simulink model "TSR_Scenario_001_cs"  (R2014b)
settings: Solver=ode5  SolverMode=SingleTasking  StartTime=0.0  StopTime=inf  FixedStep=1/100  RelTol=1e-3
PreLoadFcn:
  | mbxruntime.callbacks.PreLoadFcn(bdroot);
  | check_NUTS_defined;
  | 
  | assignin('base',['model_closed_' bdroot],false);
  | 
  | addpath('../includes_TSR/includes_TSR');
  | 
  | switch version('-release')
  | case {'2010a', '2010b', '2011a'}
  | addpath('../includes_TSR/ML2010b');
  | otherwise
  | addpath('../includes_TSR/ML2011b');
  | end
PostLoadFcn:
  | mbxruntime.callbacks.PostLoadFcn(bdroot);
InitFcn:
  | mbxruntime.callbacks.InitFcn(bdroot);
StartFcn:
  | mbxruntime.callbacks.StartFcn(bdroot);
StopFcn:
  | mbxruntime.callbacks.StopFcn(bdroot);
model workspace: external: MAT-File .\TSR_Scenario_001_cs_hws.mat (data not in the file)
undefined symbols (not defined in the file or in its folder): InitImageOutputDir, mbxruntime, OrientationPitch, OrientationRoll, PositionX, PositionY, PositionZ, tabledata, warningInitialVelocity, x0
undefined symbols (not defined in the file): SteeringColumn, SteeringWheel, TSR_Scenario_001_cs_0469e6db089af631, TSR_Scenario_001_cs_0511100212e7bc8e, TSR_Scenario_001_cs_0e7e9ae969427aac, TSR_Scenario_001_cs_1093386e49c2fe1f, TSR_Scenario_001_cs_112063adae8cf595, TSR_Scenario_001_cs_20f00d93cd5331c2, TSR_Scenario_001_cs_23e3512474fbfadc, TSR_Scenario_001_cs_366523e1554c6bf4, TSR_Scenario_001_cs_37bce4982c67337a, TSR_Scenario_001_cs_44e6164a5df50f45, TSR_Scenario_001_cs_4963ce12e7ff3247, TSR_Scenario_001_cs_4b3e01fa729ce73a, TSR_Scenario_001_cs_519c34727ce9f069, TSR_Scenario_001_cs_5b66ab60038399a1, TSR_Scenario_001_cs_5baa165dfa1afdcb, TSR_Scenario_001_cs_5f993ce39fa6372c, TSR_Scenario_001_cs_613fdf28e3ff7437, TSR_Scenario_001_cs_67b1406af835d622, TSR_Scenario_001_cs_6ad990c290286b94, TSR_Scenario_001_cs_6c412b69295984e1, TSR_Scenario_001_cs_6d4c0c06b1585ef3, TSR_Scenario_001_cs_6dd019d071bf1235, TSR_Scenario_001_cs_6e9f5883f1a78533, TSR_Scenario_001_cs_80f7223d9ac35404, TSR_Scenario_001_cs_8562b82d3c89ae57, TSR_Scenario_001_cs_8a3a0181ab0babfe, TSR_Scenario_001_cs_8c997348ce80deaf, TSR_Scenario_001_cs_925bd6a073d9fe25, TSR_Scenario_001_cs_961436216add6114, TSR_Scenario_001_cs_991a7959256b2c84, TSR_Scenario_001_cs_9a95ce2c2e753616, TSR_Scenario_001_cs_a98aa9562e8552a9, TSR_Scenario_001_cs_ab44ae81dbfb58cd, TSR_Scenario_001_cs_Actros_2541_2_Path_pathUniqueID, TSR_Scenario_001_cs_ae74836ade6bff5a, TSR_Scenario_001_cs_Audi_A8_1_Dynamics_Simple_initialPitch, TSR_Scenario_001_cs_Audi_A8_1_Dynamics_Simple_initialRoll, TSR_Scenario_001_cs_Audi_A8_1_Dynamics_Simple_initialX, TSR_Scenario_001_cs_Audi_A8_1_Dynamics_Simple_initialY, TSR_Scenario_001_cs_Audi_A8_1_Dynamics_Simple_initialYaw, TSR_Scenario_001_cs_Audi_A8_1_Dynamics_Simple_initialZ, TSR_Scenario_001_cs_Audi_A8_2_Path_pathUniqueID, TSR_Scenario_001_cs_Audi_A8_2_SpeedProfile_speedProfileUniqueID, TSR_Scenario_001_cs_b2eca4eb2fce349a, TSR_Scenario_001_cs_b7bac209c1f2549f, TSR_Scenario_001_cs_bf3dccb66d3255a4, TSR_Scenario_001_cs_bf4c1a5315e3f716, TSR_Scenario_001_cs_BMW_Z3_1_Path_pathUniqueID, TSR_Scenario_001_cs_BMW_Z3_1_SpeedProfile_speedProfileUniqueID, TSR_Scenario_001_cs_BMW_Z3_2_Path_pathUniqueID, TSR_Scenario_001_cs_BMW_Z3_2_SpeedProfile_speedProfileUniqueID, TSR_Scenario_001_cs_c4c8fc4bdece03a9, TSR_Scenario_001_cs_c964c86aa54ad92e, TSR_Scenario_001_cs_cb64d1ef85329755, TSR_Scenario_001_cs_Citroen_C3_1_Path_pathUniqueID, TSR_Scenario_001_cs_Citroen_C3_2_Path_pathUniqueID, TSR_Scenario_001_cs_Citroen_C3_3_Path_pathUniqueID, TSR_Scenario_001_cs_Citroen_C3_4_Path_pathUniqueID ... (+25)
libraries: simulink x21, PreScanSimulinkLibrary x17, simulink_extras x13
(part 16 of 30)

== system TSR_Scenario_001_cs/VISUMatrixSignLights_HighwayOverhang_6/Actuator ==
  VISUMatrixSignLights_HighwayOverhang_6 : Inport  Tag=inport/VisuMatrixSignLights  SampleTime=1/100  BusOutputAsStruct=on
  DemuxVisuLights : Demux  Outputs=16
  LimiterVisuLights : Saturate  UpperLimit=1  LowerLimit=0
  visu_MatrixSign_21_Light_1 : S-Function  FunctionName=sfun_MaterialColorSelector  Parameters=mbxruntime.parameters.convert(UniqueID), mbxruntime.parameters.convert(ColorsObjectQuery), mbxruntime.parameters.convert(Colors),tabledata, TimeStep  EnableBusSupport=off  mask(PreScan Sink Block: VisuMatrixSignLights){UniqueID=1914, ColorsObjectQuery=child:name=MatrixSign_21/child:name=HighwayOverhang_6.MatrixSign_21.OrangeLightUpperLeft, Colors=[32   25    5  255   64   48    5  255   64   54    5  255    0    0    0  255; 45   34    0  255   45   34    0  255   45   34    0  255  306  229    5  255], TimeStep=1/100}
      mask prompts: UniqueID "Parent Unique Identifier"; ColorsObjectQuery "Query for Color Object"; Colors "Matrix of colors"; TimeStep "Simulink time step"
      mask help:
      | The VisuMatrixSignLights block provides a way to switch the lights on the matrix sign board on or off
      |
      | For more information, please click Help.
      mask init:
      | [tabledata] = mbxruntime.parameters.table(UniqueID,ColorsObjectQuery,Colors);
      mask Help: eval('openHelp(732)')
      mask Display: image(imread('RearLight.png'))
  visu_MatrixSign_21_Light_2 : S-Function  FunctionName=sfun_MaterialColorSelector  Parameters=mbxruntime.parameters.convert(UniqueID), mbxruntime.parameters.convert(ColorsObjectQuery), mbxruntime.parameters.convert(Colors),tabledata, TimeStep  EnableBusSupport=off  mask(PreScan Sink Block: VisuMatrixSignLights){UniqueID=1914, ColorsObjectQuery=child:name=MatrixSign_21/child:name=HighwayOverhang_6.MatrixSign_21.OrangeLightUpperRight, Colors=[32   25    5  255   64   48    5  255   64   54    5  255    0    0    0  255; 45   34    0  255   45   34    0  255   45   34    0  255  306  229    5  255], TimeStep=1/100}
      mask prompts: UniqueID "Parent Unique Identifier"; ColorsObjectQuery "Query for Color Object"; Colors "Matrix of colors"; TimeStep "Simulink time step"
      mask help:
      | The VisuMatrixSignLights block provides a way to switch the lights on the matrix sign board on or off
      |
      | For more information, please click Help.
      mask init:
      | [tabledata] = mbxruntime.parameters.table(UniqueID,ColorsObjectQuery,Colors);
      mask Help: eval('openHelp(732)')
      mask Display: image(imread('RearLight.png'))
  visu_MatrixSign_21_Light_3 : S-Function  FunctionName=sfun_MaterialColorSelector  Parameters=mbxruntime.parameters.convert(UniqueID), mbxruntime.parameters.convert(ColorsObjectQuery), mbxruntime.parameters.convert(Colors),tabledata, TimeStep  EnableBusSupport=off  mask(PreScan Sink Block: VisuMatrixSignLights){UniqueID=1914, ColorsObjectQuery=child:name=MatrixSign_21/child:name=HighwayOverhang_6.MatrixSign_21.OrangeLightLowerLeft, Colors=[32   25    5  255   64   48    5  255   64   54    5  255    0    0    0  255; 45   34    0  255   45   34    0  255   45   34    0  255  306  229    5  255], TimeStep=1/100}
      mask prompts: UniqueID "Parent Unique Identifier"; ColorsObjectQuery "Query for Color Object"; Colors "Matrix of colors"; TimeStep "Simulink time step"
      mask help:
      | The VisuMatrixSignLights block provides a way to switch the lights on the matrix sign board on or off
      |
      | For more information, please click Help.
      mask init:
      | [tabledata] = mbxruntime.parameters.table(UniqueID,ColorsObjectQuery,Colors);
      mask Help: eval('openHelp(732)')
      mask Display: image(imread('RearLight.png'))
  visu_MatrixSign_21_Light_4 : S-Function  FunctionName=sfun_MaterialColorSelector  Parameters=mbxruntime.parameters.convert(UniqueID), mbxruntime.parameters.convert(ColorsObjectQuery), mbxruntime.parameters.convert(Colors),tabledata, TimeStep  EnableBusSupport=off  mask(PreScan Sink Block: VisuMatrixSignLights){UniqueID=1914, ColorsObjectQuery=child:name=MatrixSign_21/child:name=HighwayOverhang_6.MatrixSign_21.OrangeLightLowerRight, Colors=[32   25    5  255   64   48    5  255   64   54    5  255    0    0    0  255; 45   34    0  255   45   34    0  255   45   34    0  255  306  229    5  255], TimeStep=1/100}
      mask prompts: UniqueID "Parent Unique Identifier"; ColorsObjectQuery "Query for Color Object"; Colors "Matrix of colors"; TimeStep "Simulink time step"
      mask help:
      | The VisuMatrixSignLights block provides a way to switch the lights on the matrix sign board on or off
      |
      | For more information, please click Help.
      mask init:
      | [tabledata] = mbxruntime.parameters.table(UniqueID,ColorsObjectQuery,Colors);
      mask Help: eval('openHelp(732)')
      mask Display: image(imread('RearLight.png'))
  visu_MatrixSign_22_Light_1 : S-Function  FunctionName=sfun_MaterialColorSelector  Parameters=mbxruntime.parameters.convert(UniqueID), mbxruntime.parameters.convert(ColorsObjectQuery), mbxruntime.parameters.convert(Colors),tabledata, TimeStep  EnableBusSupport=off  mask(PreScan Sink Block: VisuMatrixSignLights){UniqueID=1914, ColorsObjectQuery=child:name=MatrixSign_22/child:name=HighwayOverhang_6.MatrixSign_22.OrangeLightUpperLeft, Colors=[32   25    5  255   64   48    5  255   64   54    5  255    0    0    0  255; 45   34    0  255   45   34    0  255   45   34    0  255  306  229    5  255], TimeStep=1/100}
      mask prompts: UniqueID "Parent Unique Identifier"; ColorsObjectQuery "Query for Color Object"; Colors "Matrix of colors"; TimeStep "Simulink time step"
      mask help:
      | The VisuMatrixSignLights block provides a way to switch the lights on the matrix sign board on or off
      |
      | For more information, please click Help.
      mask init:
      | [tabledata] = mbxruntime.parameters.table(UniqueID,ColorsObjectQuery,Colors);
      mask Help: eval('openHelp(732)')
      mask Display: image(imread('RearLight.png'))
  visu_MatrixSign_22_Light_2 : S-Function  FunctionName=sfun_MaterialColorSelector  Parameters=mbxruntime.parameters.convert(UniqueID), mbxruntime.parameters.convert(ColorsObjectQuery), mbxruntime.parameters.convert(Colors),tabledata, TimeStep  EnableBusSupport=off  mask(PreScan Sink Block: VisuMatrixSignLights){UniqueID=1914, ColorsObjectQuery=child:name=MatrixSign_22/child:name=HighwayOverhang_6.MatrixSign_22.OrangeLightUpperRight, Colors=[32   25    5  255   64   48    5  255   64   54    5  255    0    0    0  255; 45   34    0  255   45   34    0  255   45   34    0  255  306  229    5  255], TimeStep=1/100}
      mask prompts: UniqueID "Parent Unique Identifier"; ColorsObjectQuery "Query for Color Object"; Colors "Matrix of colors"; TimeStep "Simulink time step"
      mask help:
      | The VisuMatrixSignLights block provides a way to switch the lights on the matrix sign board on or off
      |
      | For more information, please click Help.
      mask init:
      | [tabledata] = mbxruntime.parameters.table(UniqueID,ColorsObjectQuery,Colors);
      mask Help: eval('openHelp(732)')
      mask Display: image(imread('RearLight.png'))
  visu_MatrixSign_22_Light_3 : S-Function  FunctionName=sfun_MaterialColorSelector  Parameters=mbxruntime.parameters.convert(UniqueID), mbxruntime.parameters.convert(ColorsObjectQuery), mbxruntime.parameters.convert(Colors),tabledata, TimeStep  EnableBusSupport=off  mask(PreScan Sink Block: VisuMatrixSignLights){UniqueID=1914, ColorsObjectQuery=child:name=MatrixSign_22/child:name=HighwayOverhang_6.MatrixSign_22.OrangeLightLowerLeft, Colors=[32   25    5  255   64   48    5  255   64   54    5  255    0    0    0  255; 45   34    0  255   45   34    0  255   45   34    0  255  306  229    5  255], TimeStep=1/100}
      mask prompts: UniqueID "Parent Unique Identifier"; ColorsObjectQuery "Query for Color Object"; Colors "Matrix of colors"; TimeStep "Simulink time step"
      mask help:
      | The VisuMatrixSignLights block provides a way to switch the lights on the matrix sign board on or off
      |
      | For more information, please click Help.
      mask init:
      | [tabledata] = mbxruntime.parameters.table(UniqueID,ColorsObjectQuery,Colors);
      mask Help: eval('openHelp(732)')
      mask Display: image(imread('RearLight.png'))
  visu_MatrixSign_22_Light_4 : S-Function  FunctionName=sfun_MaterialColorSelector  Parameters=mbxruntime.parameters.convert(UniqueID), mbxruntime.parameters.convert(ColorsObjectQuery), mbxruntime.parameters.convert(Colors),tabledata, TimeStep  EnableBusSupport=off  mask(PreScan Sink Block: VisuMatrixSignLights){UniqueID=1914, ColorsObjectQuery=child:name=MatrixSign_22/child:name=HighwayOverhang_6.MatrixSign_22.OrangeLightLowerRight, Colors=[32   25    5  255   64   48    5  255   64   54    5  255    0    0    0  255; 45   34    0  255   45   34    0  255   45   34    0  255  306  229    5  255], TimeStep=1/100}
      mask prompts: UniqueID "Parent Unique Identifier"; ColorsObjectQuery "Query for Color Object"; Colors "Matrix of colors"; TimeStep "Simulink time step"
      mask help:
      | The VisuMatrixSignLights block provides a way to switch the lights on the matrix sign board on or off
      |
      | For more information, please click Help.
      mask init:
      | [tabledata] = mbxruntime.parameters.table(UniqueID,ColorsObjectQuery,Colors);
      mask Help: eval('openHelp(732)')
      mask Display: image(imread('RearLight.png'))
  visu_MatrixSign_23_Light_1 : S-Function  FunctionName=sfun_MaterialColorSelector  Parameters=mbxruntime.parameters.convert(UniqueID), mbxruntime.parameters.convert(ColorsObjectQuery), mbxruntime.parameters.convert(Colors),tabledata, TimeStep  EnableBusSupport=off  mask(PreScan Sink Block: VisuMatrixSignLights){UniqueID=1914, ColorsObjectQuery=child:name=MatrixSign_23/child:name=HighwayOverhang_6.MatrixSign_23.OrangeLightUpperLeft, Colors=[32   25    5  255   64   48    5  255   64   54    5  255    0    0    0  255; 45   34    0  255   45   34    0  255   45   34    0  255  306  229    5  255], TimeStep=1/100}
      mask prompts: UniqueID "Parent Unique Identifier"; ColorsObjectQuery "Query for Color Object"; Colors "Matrix of colors"; TimeStep "Simulink time step"
      mask help:
      | The VisuMatrixSignLights block provides a way to switch the lights on the matrix sign board on or off
      |
      | For more information, please click Help.
      mask init:
      | [tabledata] = mbxruntime.parameters.table(UniqueID,ColorsObjectQuery,Colors);
      mask Help: eval('openHelp(732)')
      mask Display: image(imread('RearLight.png'))
  visu_MatrixSign_23_Light_2 : S-Function  FunctionName=sfun_MaterialColorSelector  Parameters=mbxruntime.parameters.convert(UniqueID), mbxruntime.parameters.convert(ColorsObjectQuery), mbxruntime.parameters.convert(Colors),tabledata, TimeStep  EnableBusSupport=off  mask(PreScan Sink Block: VisuMatrixSignLights){UniqueID=1914, ColorsObjectQuery=child:name=MatrixSign_23/child:name=HighwayOverhang_6.MatrixSign_23.OrangeLightUpperRight, Colors=[32   25    5  255   64   48    5  255   64   54    5  255    0    0    0  255; 45   34    0  255   45   34    0  255   45   34    0  255  306  229    5  255], TimeStep=1/100}
      mask prompts: UniqueID "Parent Unique Identifier"; ColorsObjectQuery "Query for Color Object"; Colors "Matrix of colors"; TimeStep "Simulink time step"
      mask help:
      | The VisuMatrixSignLights block provides a way to switch the lights on the matrix sign board on or off
      |
      | For more information, please click Help.
      mask init:
      | [tabledata] = mbxruntime.parameters.table(UniqueID,ColorsObjectQuery,Colors);
      mask Help: eval('openHelp(732)')
      mask Display: image(imread('RearLight.png'))
  visu_MatrixSign_23_Light_3 : S-Function  FunctionName=sfun_MaterialColorSelector  Parameters=mbxruntime.parameters.convert(UniqueID), mbxruntime.parameters.convert(ColorsObjectQuery), mbxruntime.parameters.convert(Colors),tabledata, TimeStep  EnableBusSupport=off  mask(PreScan Sink Block: VisuMatrixSignLights){UniqueID=1914, ColorsObjectQuery=child:name=MatrixSign_23/child:name=HighwayOverhang_6.MatrixSign_23.OrangeLightLowerLeft, Colors=[32   25    5  255   64   48    5  255   64   54    5  255    0    0    0  255; 45   34    0  255   45   34    0  255   45   34    0  255  306  229    5  255], TimeStep=1/100}
      mask prompts: UniqueID "Parent Unique Identifier"; ColorsObjectQuery "Query for Color Object"; Colors "Matrix of colors"; TimeStep "Simulink time step"
      mask help:
      | The VisuMatrixSignLights block provides a way to switch the lights on the matrix sign board on or off
      |
      | For more information, please click Help.
      mask init:
      | [tabledata] = mbxruntime.parameters.table(UniqueID,ColorsObjectQuery,Colors);
      mask Help: eval('openHelp(732)')
      mask Display: image(imread('RearLight.png'))
  visu_MatrixSign_23_Light_4 : S-Function  FunctionName=sfun_MaterialColorSelector  Parameters=mbxruntime.parameters.convert(UniqueID), mbxruntime.parameters.convert(ColorsObjectQuery), mbxruntime.parameters.convert(Colors),tabledata, TimeStep  EnableBusSupport=off  mask(PreScan Sink Block: VisuMatrixSignLights){UniqueID=1914, ColorsObjectQuery=child:name=MatrixSign_23/child:name=HighwayOverhang_6.MatrixSign_23.OrangeLightLowerRight, Colors=[32   25    5  255   64   48    5  255   64   54    5  255    0    0    0  255; 45   34    0  255   45   34    0  255   45   34    0  255  306  229    5  255], TimeStep=1/100}
      mask prompts: UniqueID "Parent Unique Identifier"; ColorsObjectQuery "Query for Color Object"; Colors "Matrix of colors"; TimeStep "Simulink time step"
      mask help:
      | The VisuMatrixSignLights block provides a way to switch the lights on the matrix sign board on or off
      |
      | For more information, please click Help.
      mask init:
      | [tabledata] = mbxruntime.parameters.table(UniqueID,ColorsObjectQuery,Colors);
      mask Help: eval('openHelp(732)')
      mask Display: image(imread('RearLight.png'))
  visu_MatrixSign_24_Light_1 : S-Function  FunctionName=sfun_MaterialColorSelector  Parameters=mbxruntime.parameters.convert(UniqueID), mbxruntime.parameters.convert(ColorsObjectQuery), mbxruntime.parameters.convert(Colors),tabledata, TimeStep  EnableBusSupport=off  mask(PreScan Sink Block: VisuMatrixSignLights){UniqueID=1914, ColorsObjectQuery=child:name=MatrixSign_24/child:name=HighwayOverhang_6.MatrixSign_24.OrangeLightUpperLeft, Colors=[32   25    5  255   64   48    5  255   64   54    5  255    0    0    0  255; 45   34    0  255   45   34    0  255   45   34    0  255  306  229    5  255], TimeStep=1/100}
      mask prompts: UniqueID "Parent Unique Identifier"; ColorsObjectQuery "Query for Color Object"; Colors "Matrix of colors"; TimeStep "Simulink time step"
      mask help:
      | The VisuMatrixSignLights block provides a way to switch the lights on the matrix sign board on or off
      |
      | For more information, please click Help.
      mask init:
      | [tabledata] = mbxruntime.parameters.table(UniqueID,ColorsObjectQuery,Colors);
      mask Help: eval('openHelp(732)')
      mask Display: image(imread('RearLight.png'))
  visu_MatrixSign_24_Light_2 : S-Function  FunctionName=sfun_MaterialColorSelector  Parameters=mbxruntime.parameters.convert(UniqueID), mbxruntime.parameters.convert(ColorsObjectQuery), mbxruntime.parameters.convert(Colors),tabledata, TimeStep  EnableBusSupport=off  mask(PreScan Sink Block: VisuMatrixSignLights){UniqueID=1914, ColorsObjectQuery=child:name=MatrixSign_24/child:name=HighwayOverhang_6.MatrixSign_24.OrangeLightUpperRight, Colors=[32   25    5  255   64   48    5  255   64   54    5  255    0    0    0  255; 45   34    0  255   45   34    0  255   45   34    0  255  306  229    5  255], TimeStep=1/100}
      mask prompts: UniqueID "Parent Unique Identifier"; ColorsObjectQuery "Query for Color Object"; Colors "Matrix of colors"; TimeStep "Simulink time step"
      mask help:
      | The VisuMatrixSignLights block provides a way to switch the lights on the matrix sign board on or off
      |
      | For more information, please click Help.
      mask init:
      | [tabledata] = mbxruntime.parameters.table(UniqueID,ColorsObjectQuery,Colors);
      mask Help: eval('openHelp(732)')
      mask Display: image(imread('RearLight.png'))
  visu_MatrixSign_24_Light_3 : S-Function  FunctionName=sfun_MaterialColorSelector  Parameters=mbxruntime.parameters.convert(UniqueID), mbxruntime.parameters.convert(ColorsObjectQuery), mbxruntime.parameters.convert(Colors),tabledata, TimeStep  EnableBusSupport=off  mask(PreScan Sink Block: VisuMatrixSignLights){UniqueID=1914, ColorsObjectQuery=child:name=MatrixSign_24/child:name=HighwayOverhang_6.MatrixSign_24.OrangeLightLowerLeft, Colors=[32   25    5  255   64   48    5  255   64   54    5  255    0    0    0  255; 45   34    0  255   45   34    0  255   45   34    0  255  306  229    5  255], TimeStep=1/100}
      mask prompts: UniqueID "Parent Unique Identifier"; ColorsObjectQuery "Query for Color Object"; Colors "Matrix of colors"; TimeStep "Simulink time step"
      mask help:
      | The VisuMatrixSignLights block provides a way to switch the lights on the matrix sign board on or off
      |
      | For more information, please click Help.
      mask init:
      | [tabledata] = mbxruntime.parameters.table(UniqueID,ColorsObjectQuery,Colors);
      mask Help: eval('openHelp(732)')
      mask Display: image(imread('RearLight.png'))
  visu_MatrixSign_24_Light_4 : S-Function  FunctionName=sfun_MaterialColorSelector  Parameters=mbxruntime.parameters.convert(UniqueID), mbxruntime.parameters.convert(ColorsObjectQuery), mbxruntime.parameters.convert(Colors),tabledata, TimeStep  EnableBusSupport=off  mask(PreScan Sink Block: VisuMatrixSignLights){UniqueID=1914, ColorsObjectQuery=child:name=MatrixSign_24/child:name=HighwayOverhang_6.MatrixSign_24.OrangeLightLowerRight, Colors=[32   25    5  255   64   48    5  255   64   54    5  255    0    0    0  255; 45   34    0  255   45   34    0  255   45   34    0  255  306  229    5  255], TimeStep=1/100}
      mask prompts: UniqueID "Parent Unique Identifier"; ColorsObjectQuery "Query for Color Object"; Colors "Matrix of colors"; TimeStep "Simulink time step"
      mask help:
      | The VisuMatrixSignLights block provides a way to switch the lights on the matrix sign board on or off
      |
      | For more information, please click Help.
      mask init:
      | [tabledata] = mbxruntime.parameters.table(UniqueID,ColorsObjectQuery,Colors);
      mask Help: eval('openHelp(732)')
      mask Display: image(imread('RearLight.png'))
  wires:
  VISUMatrixSignLights_HighwayOverhang_6/1 -> LimiterVisuLights/1
  LimiterVisuLights/1 -> DemuxVisuLights/1
  DemuxVisuLights/1 -> visu_MatrixSign_21_Light_1/1
  DemuxVisuLights/2 -> visu_MatrixSign_21_Light_2/1
  DemuxVisuLights/3 -> visu_MatrixSign_21_Light_3/1
  DemuxVisuLights/4 -> visu_MatrixSign_21_Light_4/1
  DemuxVisuLights/5 -> visu_MatrixSign_22_Light_1/1
  DemuxVisuLights/6 -> visu_MatrixSign_22_Light_2/1
  DemuxVisuLights/7 -> visu_MatrixSign_22_Light_3/1
  DemuxVisuLights/8 -> visu_MatrixSign_22_Light_4/1
  DemuxVisuLights/9 -> visu_MatrixSign_23_Light_1/1
  DemuxVisuLights/10 -> visu_MatrixSign_23_Light_2/1
  DemuxVisuLights/11 -> visu_MatrixSign_23_Light_3/1
  DemuxVisuLights/12 -> visu_MatrixSign_23_Light_4/1
  DemuxVisuLights/13 -> visu_MatrixSign_24_Light_1/1
  DemuxVisuLights/14 -> visu_MatrixSign_24_Light_2/1
  DemuxVisuLights/15 -> visu_MatrixSign_24_Light_3/1
  DemuxVisuLights/16 -> visu_MatrixSign_24_Light_4/1

== system TSR_Scenario_001_cs/VISUMatrixSign_HighwayOverhang_1/Actuator ==
  VISUMatrixSign_HighwayOverhang_1 : Inport  Tag=inport/VisuMatrixSign  SampleTime=1/100  BusOutputAsStruct=on
  DemuxVisuMatrixSign : Demux
  visu_MatrixSign_1 : S-Function  FunctionName=sfun_ResourceNameSelector  Parameters=mbxruntime.parameters.convert(UniqueID), mbxruntime.parameters.convert(ResourceList), mbxruntime.parameters.convert(PivotName),tabledata, TimeStep  EnableBusSupport=off  mask(PreScan Sink Block: VisuMatrixSign){UniqueID=1876, ResourceList={'3' 'InformationSign\MatrixSign_Empty.png' '4' 'InformationSign\MatrixSign_End.png' '5' 'InformationSign\MatrixSign_GreenArrow.png' '6' 'InformationSign\MatrixSign_RedCross.png' '7' 'InformationSign\MatrixSign_Speed_50.png' '8' 'InformationSign\MatrixSign_Speed_70.png' '9' 'InformationSign\MatrixSign_Speed_90.png' '10' 'InformationSign\MatrixSign_Speed_120.png' '11' 'InformationSign\MatrixSign_Speed_130.png' '12' 'InformationSign\information.png' '13' 'InformationSign\Empty.jpg' }, PivotName=/child:name=MatrixSign_1/trafficSignElement, TimeStep=1/100}
      mask prompts: UniqueID "Parent Unique Identifier (auto-generated)"; ResourceList "Resource List (auto-generated)"; PivotName "Name of pivot (auto-generated)"; TimeStep "Simulink time step"
      mask help:
      | The VisuMatrixSign block provides a way to adapt the texture of the plates connected to an overhang, based on Resource IDs of the texture files.
      |
      | For more information, please click Help.
      mask init:
      | [tabledata] = mbxruntime.parameters.table(UniqueID,ResourceList,PivotName);
      mask Help: eval('openHelp(733)')
      mask Display: image(imread('HighwaySpeedMatrix.png'))
  visu_MatrixSign_2 : S-Function  FunctionName=sfun_ResourceNameSelector  Parameters=mbxruntime.parameters.convert(UniqueID), mbxruntime.parameters.convert(ResourceList), mbxruntime.parameters.convert(PivotName),tabledata, TimeStep  EnableBusSupport=off  mask(PreScan Sink Block: VisuMatrixSign){UniqueID=1876, ResourceList={'3' 'InformationSign\MatrixSign_Empty.png' '4' 'InformationSign\MatrixSign_End.png' '5' 'InformationSign\MatrixSign_GreenArrow.png' '6' 'InformationSign\MatrixSign_RedCross.png' '7' 'InformationSign\MatrixSign_Speed_50.png' '8' 'InformationSign\MatrixSign_Speed_70.png' '9' 'InformationSign\MatrixSign_Speed_90.png' '10' 'InformationSign\MatrixSign_Speed_120.png' '11' 'InformationSign\MatrixSign_Speed_130.png' '12' 'InformationSign\information.png' '13' 'InformationSign\Empty.jpg' }, PivotName=/child:name=MatrixSign_2/trafficSignElement, TimeStep=1/100}
      mask prompts: UniqueID "Parent Unique Identifier (auto-generated)"; ResourceList "Resource List (auto-generated)"; PivotName "Name of pivot (auto-generated)"; TimeStep "Simulink time step"
      mask help:
      | The VisuMatrixSign block provides a way to adapt the texture of the plates connected to an overhang, based on Resource IDs of the texture files.
      |
      | For more information, please click Help.
      mask init:
      | [tabledata] = mbxruntime.parameters.table(UniqueID,ResourceList,PivotName);
      mask Help: eval('openHelp(733)')
      mask Display: image(imread('HighwaySpeedMatrix.png'))
  visu_MatrixSign_3 : S-Function  FunctionName=sfun_ResourceNameSelector  Parameters=mbxruntime.parameters.convert(UniqueID), mbxruntime.parameters.convert(ResourceList), mbxruntime.parameters.convert(PivotName),tabledata, TimeStep  EnableBusSupport=off  mask(PreScan Sink Block: VisuMatrixSign){UniqueID=1876, ResourceList={'3' 'InformationSign\MatrixSign_Empty.png' '4' 'InformationSign\MatrixSign_End.png' '5' 'InformationSign\MatrixSign_GreenArrow.png' '6' 'InformationSign\MatrixSign_RedCross.png' '7' 'InformationSign\MatrixSign_Speed_50.png' '8' 'InformationSign\MatrixSign_Speed_70.png' '9' 'InformationSign\MatrixSign_Speed_90.png' '10' 'InformationSign\MatrixSign_Speed_120.png' '11' 'InformationSign\MatrixSign_Speed_130.png' '12' 'InformationSign\information.png' '13' 'InformationSign\Empty.jpg' }, PivotName=/child:name=MatrixSign_3/trafficSignElement, TimeStep=1/100}
      mask prompts: UniqueID "Parent Unique Identifier (auto-generated)"; ResourceList "Resource List (auto-generated)"; PivotName "Name of pivot (auto-generated)"; TimeStep "Simulink time step"
      mask help:
      | The VisuMatrixSign block provides a way to adapt the texture of the plates connected to an overhang, based on Resource IDs of the texture files.
      |
      | For more information, please click Help.
      mask init:
      | [tabledata] = mbxruntime.parameters.table(UniqueID,ResourceList,PivotName);
      mask Help: eval('openHelp(733)')
      mask Display: image(imread('HighwaySpeedMatrix.png'))
  visu_MatrixSign_4 : S-Function  FunctionName=sfun_ResourceNameSelector  Parameters=mbxruntime.parameters.convert(UniqueID), mbxruntime.parameters.convert(ResourceList), mbxruntime.parameters.convert(PivotName),tabledata, TimeStep  EnableBusSupport=off  mask(PreScan Sink Block: VisuMatrixSign){UniqueID=1876, ResourceList={'3' 'InformationSign\MatrixSign_Empty.png' '4' 'InformationSign\MatrixSign_End.png' '5' 'InformationSign\MatrixSign_GreenArrow.png' '6' 'InformationSign\MatrixSign_RedCross.png' '7' 'InformationSign\MatrixSign_Speed_50.png' '8' 'InformationSign\MatrixSign_Speed_70.png' '9' 'InformationSign\MatrixSign_Speed_90.png' '10' 'InformationSign\MatrixSign_Speed_120.png' '11' 'InformationSign\MatrixSign_Speed_130.png' '12' 'InformationSign\information.png' '13' 'InformationSign\Empty.jpg' }, PivotName=/child:name=MatrixSign_4/trafficSignElement, TimeStep=1/100}
      mask prompts: UniqueID "Parent Unique Identifier (auto-generated)"; ResourceList "Resource List (auto-generated)"; PivotName "Name of pivot (auto-generated)"; TimeStep "Simulink time step"
      mask help:
      | The VisuMatrixSign block provides a way to adapt the texture of the plates connected to an overhang, based on Resource IDs of the texture files.
      |
      | For more information, please click Help.
      mask init:
      | [tabledata] = mbxruntime.parameters.table(UniqueID,ResourceList,PivotName);
      mask Help: eval('openHelp(733)')
      mask Display: image(imread('HighwaySpeedMatrix.png'))
  wires:
  VISUMatrixSign_HighwayOverhang_1/1 -> DemuxVisuMatrixSign/1
  DemuxVisuMatrixSign/1 -> visu_MatrixSign_1/1
  DemuxVisuMatrixSign/2 -> visu_MatrixSign_2/1
  DemuxVisuMatrixSign/3 -> visu_MatrixSign_3/1
  DemuxVisuMatrixSign/4 -> visu_MatrixSign_4/1

== system TSR_Scenario_001_cs/VISUMatrixSign_HighwayOverhang_2/Actuator ==
  VISUMatrixSign_HighwayOverhang_2 : Inport  Tag=inport/VisuMatrixSign  SampleTime=1/100  BusOutputAsStruct=on
  DemuxVisuMatrixSign : Demux
  visu_MatrixSign_5 : S-Function  FunctionName=sfun_ResourceNameSelector  Parameters=mbxruntime.parameters.convert(UniqueID), mbxruntime.parameters.convert(ResourceList), mbxruntime.parameters.convert(PivotName),tabledata, TimeStep  EnableBusSupport=off  mask(PreScan Sink Block: VisuMatrixSign){UniqueID=1877, ResourceList={'3' 'InformationSign\MatrixSign_Empty.png' '4' 'InformationSign\MatrixSign_End.png' '5' 'InformationSign\MatrixSign_GreenArrow.png' '6' 'InformationSign\MatrixSign_RedCross.png' '7' 'InformationSign\MatrixSign_Speed_50.png' '8' 'InformationSign\MatrixSign_Speed_70.png' '9' 'InformationSign\MatrixSign_Speed_90.png' '10' 'InformationSign\MatrixSign_Speed_120.png' '11' 'InformationSign\MatrixSign_Speed_130.png' '12' 'InformationSign\information.png' '13' 'InformationSign\Empty.jpg' }, PivotName=/child:name=MatrixSign_5/trafficSignElement, TimeStep=1/100}
      mask prompts: UniqueID "Parent Unique Identifier (auto-generated)"; ResourceList "Resource List (auto-generated)"; PivotName "Name of pivot (auto-generated)"; TimeStep "Simulink time step"
      mask help:
      | The VisuMatrixSign block provides a way to adapt the texture of the plates connected to an overhang, based on Resource IDs of the texture files.
      |
      | For more information, please click Help.
      mask init:
      | [tabledata] = mbxruntime.parameters.table(UniqueID,ResourceList,PivotName);
      mask Help: eval('openHelp(733)')
      mask Display: image(imread('HighwaySpeedMatrix.png'))
  visu_MatrixSign_6 : S-Function  FunctionName=sfun_ResourceNameSelector  Parameters=mbxruntime.parameters.convert(UniqueID), mbxruntime.parameters.convert(ResourceList), mbxruntime.parameters.convert(PivotName),tabledata, TimeStep  EnableBusSupport=off  mask(PreScan Sink Block: VisuMatrixSign){UniqueID=1877, ResourceList={'3' 'InformationSign\MatrixSign_Empty.png' '4' 'InformationSign\MatrixSign_End.png' '5' 'InformationSign\MatrixSign_GreenArrow.png' '6' 'InformationSign\MatrixSign_RedCross.png' '7' 'InformationSign\MatrixSign_Speed_50.png' '8' 'InformationSign\MatrixSign_Speed_70.png' '9' 'InformationSign\MatrixSign_Speed_90.png' '10' 'InformationSign\MatrixSign_Speed_120.png' '11' 'InformationSign\MatrixSign_Speed_130.png' '12' 'InformationSign\information.png' '13' 'InformationSign\Empty.jpg' }, PivotName=/child:name=MatrixSign_6/trafficSignElement, TimeStep=1/100}
      mask prompts: UniqueID "Parent Unique Identifier (auto-generated)"; ResourceList "Resource List (auto-generated)"; PivotName "Name of pivot (auto-generated)"; TimeStep "Simulink time step"
      mask help:
      | The VisuMatrixSign block provides a way to adapt the texture of the plates connected to an overhang, based on Resource IDs of the texture files.
      |
      | For more information, please click Help.
      mask init:
      | [tabledata] = mbxruntime.parameters.table(UniqueID,ResourceList,PivotName);
      mask Help: eval('openHelp(733)')
      mask Display: image(imread('HighwaySpeedMatrix.png'))
  visu_MatrixSign_7 : S-Function  FunctionName=sfun_ResourceNameSelector  Parameters=mbxruntime.parameters.convert(UniqueID), mbxruntime.parameters.convert(ResourceList), mbxruntime.parameters.convert(PivotName),tabledata, TimeStep  EnableBusSupport=off  mask(PreScan Sink Block: VisuMatrixSign){UniqueID=1877, ResourceList={'3' 'InformationSign\MatrixSign_Empty.png' '4' 'InformationSign\MatrixSign_End.png' '5' 'InformationSign\MatrixSign_GreenArrow.png' '6' 'InformationSign\MatrixSign_RedCross.png' '7' 'InformationSign\MatrixSign_Speed_50.png' '8' 'InformationSign\MatrixSign_Speed_70.png' '9' 'InformationSign\MatrixSign_Speed_90.png' '10' 'InformationSign\MatrixSign_Speed_120.png' '11' 'InformationSign\MatrixSign_Speed_130.png' '12' 'InformationSign\information.png' '13' 'InformationSign\Empty.jpg' }, PivotName=/child:name=MatrixSign_7/trafficSignElement, TimeStep=1/100}
      mask prompts: UniqueID "Parent Unique Identifier (auto-generated)"; ResourceList "Resource List (auto-generated)"; PivotName "Name of pivot (auto-generated)"; TimeStep "Simulink time step"
      mask help:
      | The VisuMatrixSign block provides a way to adapt the texture of the plates connected to an overhang, based on Resource IDs of the texture files.
      |
      | For more information, please click Help.
      mask init:
      | [tabledata] = mbxruntime.parameters.table(UniqueID,ResourceList,PivotName);
      mask Help: eval('openHelp(733)')
      mask Display: image(imread('HighwaySpeedMatrix.png'))
  visu_MatrixSign_8 : S-Function  FunctionName=sfun_ResourceNameSelector  Parameters=mbxruntime.parameters.convert(UniqueID), mbxruntime.parameters.convert(ResourceList), mbxruntime.parameters.convert(PivotName),tabledata, TimeStep  EnableBusSupport=off  mask(PreScan Sink Block: VisuMatrixSign){UniqueID=1877, ResourceList={'3' 'InformationSign\MatrixSign_Empty.png' '4' 'InformationSign\MatrixSign_End.png' '5' 'InformationSign\MatrixSign_GreenArrow.png' '6' 'InformationSign\MatrixSign_RedCross.png' '7' 'InformationSign\MatrixSign_Speed_50.png' '8' 'InformationSign\MatrixSign_Speed_70.png' '9' 'InformationSign\MatrixSign_Speed_90.png' '10' 'InformationSign\MatrixSign_Speed_120.png' '11' 'InformationSign\MatrixSign_Speed_130.png' '12' 'InformationSign\information.png' '13' 'InformationSign\Empty.jpg' }, PivotName=/child:name=MatrixSign_8/trafficSignElement, TimeStep=1/100}
      mask prompts: UniqueID "Parent Unique Identifier (auto-generated)"; ResourceList "Resource List (auto-generated)"; PivotName "Name of pivot (auto-generated)"; TimeStep "Simulink time step"
      mask help:
      | The VisuMatrixSign block provides a way to adapt the texture of the plates connected to an overhang, based on Resource IDs of the texture files.
      |
      | For more information, please click Help.
      mask init:
      | [tabledata] = mbxruntime.parameters.table(UniqueID,ResourceList,PivotName);
      mask Help: eval('openHelp(733)')
      mask Display: image(imread('HighwaySpeedMatrix.png'))
  wires:
  VISUMatrixSign_HighwayOverhang_2/1 -> DemuxVisuMatrixSign/1
  DemuxVisuMatrixSign/1 -> visu_MatrixSign_5/1
  DemuxVisuMatrixSign/2 -> visu_MatrixSign_6/1
  DemuxVisuMatrixSign/3 -> visu_MatrixSign_7/1
  DemuxVisuMatrixSign/4 -> visu_MatrixSign_8/1

== system TSR_Scenario_001_cs/VISUMatrixSign_HighwayOverhang_3/Actuator ==
  VISUMatrixSign_HighwayOverhang_3 : Inport  Tag=inport/VisuMatrixSign  SampleTime=1/100  BusOutputAsStruct=on
  DemuxVisuMatrixSign : Demux
  visu_MatrixSign_10 : S-Function  FunctionName=sfun_ResourceNameSelector  Parameters=mbxruntime.parameters.convert(UniqueID), mbxruntime.parameters.convert(ResourceList), mbxruntime.parameters.convert(PivotName),tabledata, TimeStep  EnableBusSupport=off  mask(PreScan Sink Block: VisuMatrixSign){UniqueID=1890, ResourceList={'3' 'InformationSign\MatrixSign_Empty.png' '4' 'InformationSign\MatrixSign_End.png' '5' 'InformationSign\MatrixSign_GreenArrow.png' '6' 'InformationSign\MatrixSign_RedCross.png' '7' 'InformationSign\MatrixSign_Speed_50.png' '8' 'InformationSign\MatrixSign_Speed_70.png' '9' 'InformationSign\MatrixSign_Speed_90.png' '10' 'InformationSign\MatrixSign_Speed_120.png' '11' 'InformationSign\MatrixSign_Speed_130.png' '12' 'InformationSign\information.png' '13' 'InformationSign\Empty.jpg' }, PivotName=/child:name=MatrixSign_10/trafficSignElement, TimeStep=1/100}
      mask prompts: UniqueID "Parent Unique Identifier (auto-generated)"; ResourceList "Resource List (auto-generated)"; PivotName "Name of pivot (auto-generated)"; TimeStep "Simulink time step"
      mask help:
      | The VisuMatrixSign block provides a way to adapt the texture of the plates connected to an overhang, based on Resource IDs of the texture files.
      |
      | For more information, please click Help.
      mask init:
      | [tabledata] = mbxruntime.parameters.table(UniqueID,ResourceList,PivotName);
      mask Help: eval('openHelp(733)')
      mask Display: image(imread('HighwaySpeedMatrix.png'))
  visu_MatrixSign_11 : S-Function  FunctionName=sfun_ResourceNameSelector  Parameters=mbxruntime.parameters.convert(UniqueID), mbxruntime.parameters.convert(ResourceList), mbxruntime.parameters.convert(PivotName),tabledata, TimeStep  EnableBusSupport=off  mask(PreScan Sink Block: VisuMatrixSign){UniqueID=1890, ResourceList={'3' 'InformationSign\MatrixSign_Empty.png' '4' 'InformationSign\MatrixSign_End.png' '5' 'InformationSign\MatrixSign_GreenArrow.png' '6' 'InformationSign\MatrixSign_RedCross.png' '7' 'InformationSign\MatrixSign_Speed_50.png' '8' 'InformationSign\MatrixSign_Speed_70.png' '9' 'InformationSign\MatrixSign_Speed_90.png' '10' 'InformationSign\MatrixSign_Speed_120.png' '11' 'InformationSign\MatrixSign_Speed_130.png' '12' 'InformationSign\information.png' '13' 'InformationSign\Empty.jpg' }, PivotName=/child:name=MatrixSign_11/trafficSignElement, TimeStep=1/100}
      mask prompts: UniqueID "Parent Unique Identifier (auto-generated)"; ResourceList "Resource List (auto-generated)"; PivotName "Name of pivot (auto-generated)"; TimeStep "Simulink time step"
      mask help:
      | The VisuMatrixSign block provides a way to adapt the texture of the plates connected to an overhang, based on Resource IDs of the texture files.
      |
      | For more information, please click Help.
      mask init:
      | [tabledata] = mbxruntime.parameters.table(UniqueID,ResourceList,PivotName);
      mask Help: eval('openHelp(733)')
      mask Display: image(imread('HighwaySpeedMatrix.png'))
  visu_MatrixSign_12 : S-Function  FunctionName=sfun_ResourceNameSelector  Parameters=mbxruntime.parameters.convert(UniqueID), mbxruntime.parameters.convert(ResourceList), mbxruntime.parameters.convert(PivotName),tabledata, TimeStep  EnableBusSupport=off  mask(PreScan Sink Block: VisuMatrixSign){UniqueID=1890, ResourceList={'3' 'InformationSign\MatrixSign_Empty.png' '4' 'InformationSign\MatrixSign_End.png' '5' 'InformationSign\MatrixSign_GreenArrow.png' '6' 'InformationSign\MatrixSign_RedCross.png' '7' 'InformationSign\MatrixSign_Speed_50.png' '8' 'InformationSign\MatrixSign_Speed_70.png' '9' 'InformationSign\MatrixSign_Speed_90.png' '10' 'InformationSign\MatrixSign_Speed_120.png' '11' 'InformationSign\MatrixSign_Speed_130.png' '12' 'InformationSign\information.png' '13' 'InformationSign\Empty.jpg' }, PivotName=/child:name=MatrixSign_12/trafficSignElement, TimeStep=1/100}
      mask prompts: UniqueID "Parent Unique Identifier (auto-generated)"; ResourceList "Resource List (auto-generated)"; PivotName "Name of pivot (auto-generated)"; TimeStep "Simulink time step"
      mask help:
      | The VisuMatrixSign block provides a way to adapt the texture of the plates connected to an overhang, based on Resource IDs of the texture files.
      |
      | For more information, please click Help.
      mask init:
      | [tabledata] = mbxruntime.parameters.table(UniqueID,ResourceList,PivotName);
      mask Help: eval('openHelp(733)')
      mask Display: image(imread('HighwaySpeedMatrix.png'))
  visu_MatrixSign_9 : S-Function  FunctionName=sfun_ResourceNameSelector  Parameters=mbxruntime.parameters.convert(UniqueID), mbxruntime.parameters.convert(ResourceList), mbxruntime.parameters.convert(PivotName),tabledata, TimeStep  EnableBusSupport=off  mask(PreScan Sink Block: VisuMatrixSign){UniqueID=1890, ResourceList={'3' 'InformationSign\MatrixSign_Empty.png' '4' 'InformationSign\MatrixSign_End.png' '5' 'InformationSign\MatrixSign_GreenArrow.png' '6' 'InformationSign\MatrixSign_RedCross.png' '7' 'InformationSign\MatrixSign_Speed_50.png' '8' 'InformationSign\MatrixSign_Speed_70.png' '9' 'InformationSign\MatrixSign_Speed_90.png' '10' 'InformationSign\MatrixSign_Speed_120.png' '11' 'InformationSign\MatrixSign_Speed_130.png' '12' 'InformationSign\information.png' '13' 'InformationSign\Empty.jpg' }, PivotName=/child:name=MatrixSign_9/trafficSignElement, TimeStep=1/100}
      mask prompts: UniqueID "Parent Unique Identifier (auto-generated)"; ResourceList "Resource List (auto-generated)"; PivotName "Name of pivot (auto-generated)"; TimeStep "Simulink time step"
      mask help:
      | The VisuMatrixSign block provides a way to adapt the texture of the plates connected to an overhang, based on Resource IDs of the texture files.
      |
      | For more information, please click Help.
      mask init:
      | [tabledata] = mbxruntime.parameters.table(UniqueID,ResourceList,PivotName);
      mask Help: eval('openHelp(733)')
      mask Display: image(imread('HighwaySpeedMatrix.png'))
  wires:
  VISUMatrixSign_HighwayOverhang_3/1 -> DemuxVisuMatrixSign/1
  DemuxVisuMatrixSign/1 -> visu_MatrixSign_9/1
  DemuxVisuMatrixSign/2 -> visu_MatrixSign_10/1
  DemuxVisuMatrixSign/3 -> visu_MatrixSign_11/1
  DemuxVisuMatrixSign/4 -> visu_MatrixSign_12/1

== system TSR_Scenario_001_cs/VISUMatrixSign_HighwayOverhang_4/Actuator ==
  VISUMatrixSign_HighwayOverhang_4 : Inport  Tag=inport/VisuMatrixSign  SampleTime=1/100  BusOutputAsStruct=on
  DemuxVisuMatrixSign : Demux
  visu_MatrixSign_13 : S-Function  FunctionName=sfun_ResourceNameSelector  Parameters=mbxruntime.parameters.convert(UniqueID), mbxruntime.parameters.convert(ResourceList), mbxruntime.parameters.convert(PivotName),tabledata, TimeStep  EnableBusSupport=off  mask(PreScan Sink Block: VisuMatrixSign){UniqueID=1898, ResourceList={'3' 'InformationSign\MatrixSign_Empty.png' '4' 'InformationSign\MatrixSign_End.png' '5' 'InformationSign\MatrixSign_GreenArrow.png' '6' 'InformationSign\MatrixSign_RedCross.png' '7' 'InformationSign\MatrixSign_Speed_50.png' '8' 'InformationSign\MatrixSign_Speed_70.png' '9' 'InformationSign\MatrixSign_Speed_90.png' '10' 'InformationSign\MatrixSign_Speed_120.png' '11' 'InformationSign\MatrixSign_Speed_130.png' '12' 'InformationSign\information.png' '13' 'InformationSign\Empty.jpg' }, PivotName=/child:name=MatrixSign_13/trafficSignElement, TimeStep=1/100}
      mask prompts: UniqueID "Parent Unique Identifier (auto-generated)"; ResourceList "Resource List (auto-generated)"; PivotName "Name of pivot (auto-generated)"; TimeStep "Simulink time step"
      mask help:
      | The VisuMatrixSign block provides a way to adapt the texture of the plates connected to an overhang, based on Resource IDs of the texture files.
      |
      | For more information, please click Help.
      mask init:
      | [tabledata] = mbxruntime.parameters.table(UniqueID,ResourceList,PivotName);
      mask Help: eval('openHelp(733)')
      mask Display: image(imread('HighwaySpeedMatrix.png'))
  visu_MatrixSign_14 : S-Function  FunctionName=sfun_ResourceNameSelector  Parameters=mbxruntime.parameters.convert(UniqueID), mbxruntime.parameters.convert(ResourceList), mbxruntime.parameters.convert(PivotName),tabledata, TimeStep  EnableBusSupport=off  mask(PreScan Sink Block: VisuMatrixSign){UniqueID=1898, ResourceList={'3' 'InformationSign\MatrixSign_Empty.png' '4' 'InformationSign\MatrixSign_End.png' '5' 'InformationSign\MatrixSign_GreenArrow.png' '6' 'InformationSign\MatrixSign_RedCross.png' '7' 'InformationSign\MatrixSign_Speed_50.png' '8' 'InformationSign\MatrixSign_Speed_70.png' '9' 'InformationSign\MatrixSign_Speed_90.png' '10' 'InformationSign\MatrixSign_Speed_120.png' '11' 'InformationSign\MatrixSign_Speed_130.png' '12' 'InformationSign\information.png' '13' 'InformationSign\Empty.jpg' }, PivotName=/child:name=MatrixSign_14/trafficSignElement, TimeStep=1/100}
      mask prompts: UniqueID "Parent Unique Identifier (auto-generated)"; ResourceList "Resource List (auto-generated)"; PivotName "Name of pivot (auto-generated)"; TimeStep "Simulink time step"
      mask help:
      | The VisuMatrixSign block provides a way to adapt the texture of the plates connected to an overhang, based on Resource IDs of the texture files.
      |
      | For more information, please click Help.
      mask init:
      | [tabledata] = mbxruntime.parameters.table(UniqueID,ResourceList,PivotName);
      mask Help: eval('openHelp(733)')
      mask Display: image(imread('HighwaySpeedMatrix.png'))
  visu_MatrixSign_15 : S-Function  FunctionName=sfun_ResourceNameSelector  Parameters=mbxruntime.parameters.convert(UniqueID), mbxruntime.parameters.convert(ResourceList), mbxruntime.parameters.convert(PivotName),tabledata, TimeStep  EnableBusSupport=off  mask(PreScan Sink Block: VisuMatrixSign){UniqueID=1898, ResourceList={'3' 'InformationSign\MatrixSign_Empty.png' '4' 'InformationSign\MatrixSign_End.png' '5' 'InformationSign\MatrixSign_GreenArrow.png' '6' 'InformationSign\MatrixSign_RedCross.png' '7' 'InformationSign\MatrixSign_Speed_50.png' '8' 'InformationSign\MatrixSign_Speed_70.png' '9' 'InformationSign\MatrixSign_Speed_90.png' '10' 'InformationSign\MatrixSign_Speed_120.png' '11' 'InformationSign\MatrixSign_Speed_130.png' '12' 'InformationSign\information.png' '13' 'InformationSign\Empty.jpg' }, PivotName=/child:name=MatrixSign_15/trafficSignElement, TimeStep=1/100}
      mask prompts: UniqueID "Parent Unique Identifier (auto-generated)"; ResourceList "Resource List (auto-generated)"; PivotName "Name of pivot (auto-generated)"; TimeStep "Simulink time step"
      mask help:
      | The VisuMatrixSign block provides a way to adapt the texture of the plates connected to an overhang, based on Resource IDs of the texture files.
      |
      | For more information, please click Help.
      mask init:
      | [tabledata] = mbxruntime.parameters.table(UniqueID,ResourceList,PivotName);
      mask Help: eval('openHelp(733)')
      mask Display: image(imread('HighwaySpeedMatrix.png'))
  visu_MatrixSign_16 : S-Function  FunctionName=sfun_ResourceNameSelector  Parameters=mbxruntime.parameters.convert(UniqueID), mbxruntime.parameters.convert(ResourceList), mbxruntime.parameters.convert(PivotName),tabledata, TimeStep  EnableBusSupport=off  mask(PreScan Sink Block: VisuMatrixSign){UniqueID=1898, ResourceList={'3' 'InformationSign\MatrixSign_Empty.png' '4' 'InformationSign\MatrixSign_End.png' '5' 'InformationSign\MatrixSign_GreenArrow.png' '6' 'InformationSign\MatrixSign_RedCross.png' '7' 'InformationSign\MatrixSign_Speed_50.png' '8' 'InformationSign\MatrixSign_Speed_70.png' '9' 'InformationSign\MatrixSign_Speed_90.png' '10' 'InformationSign\MatrixSign_Speed_120.png' '11' 'InformationSign\MatrixSign_Speed_130.png' '12' 'InformationSign\information.png' '13' 'InformationSign\Empty.jpg' }, PivotName=/child:name=MatrixSign_16/trafficSignElement, TimeStep=1/100}
      mask prompts: UniqueID "Parent Unique Identifier (auto-generated)"; ResourceList "Resource List (auto-generated)"; PivotName "Name of pivot (auto-generated)"; TimeStep "Simulink time step"
      mask help:
      | The VisuMatrixSign block provides a way to adapt the texture of the plates connected to an overhang, based on Resource IDs of the texture files.
      |
      | For more information, please click Help.
      mask init:
      | [tabledata] = mbxruntime.parameters.table(UniqueID,ResourceList,PivotName);
      mask Help: eval('openHelp(733)')
      mask Display: image(imread('HighwaySpeedMatrix.png'))
  wires:
  VISUMatrixSign_HighwayOverhang_4/1 -> DemuxVisuMatrixSign/1
  DemuxVisuMatrixSign/1 -> visu_MatrixSign_13/1
  DemuxVisuMatrixSign/2 -> visu_MatrixSign_14/1
  DemuxVisuMatrixSign/3 -> visu_MatrixSign_15/1
  DemuxVisuMatrixSign/4 -> visu_MatrixSign_16/1
